simulink library "SADlibrary"  (R2020b)
settings: Solver=VariableStepAuto  StartTime=0.0  StopTime=10.0  RelTol=1e-3
libraries: vrlib x1, aerolibutil x1
settings Model: Creator=matteo  LastModifiedBy=matteo

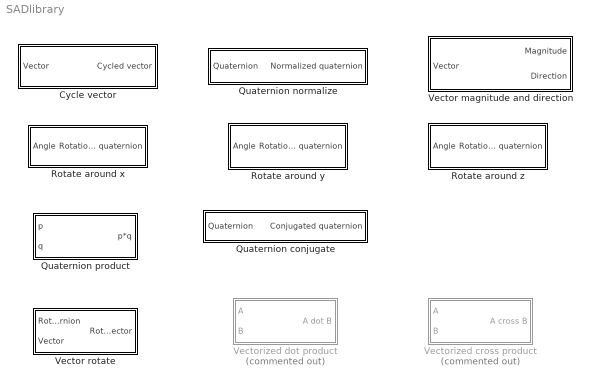
== system SADlibrary ==
  Cycle vector : Subsystem
  Quaternion conjugate : Subsystem
  Quaternion normalize : Subsystem
  Quaternion product : Subsystem
  Rotate around x : Subsystem
  Rotate around y : Subsystem
  Rotate around z : Subsystem
  Vector magnitude and direction : Subsystem
  Vector rotate : Subsystem
  Vectorized cross product : Subsystem  Commented=on
  Vectorized dot product : Subsystem  Commented=on

== system SADlibrary/Cycle vector ==
  Vector : Inport
  Demux : Demux  Outputs=2
  Mux : Mux  Inputs=2
  Cycled vector : Outport
  wires:
  Demux/1 -> Mux/2
  Mux/1 -> Cycled vector/1
  Vector/1 -> Demux/1
  Demux/2 -> Mux/1

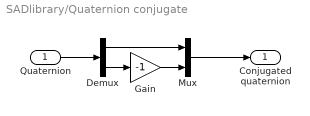
== system SADlibrary/Quaternion conjugate ==
  Quaternion : Inport
  Demux : Demux  Outputs=2
  Gain : Gain  Gain=-1
  Mux : Mux  Inputs=2
  Conjugated quaternion : Outport
  wires:
  Quaternion/1 -> Demux/1
  Demux/2 -> Gain/1
  Gain/1 -> Mux/2
  Demux/1 -> Mux/1
  Mux/1 -> Conjugated quaternion/1

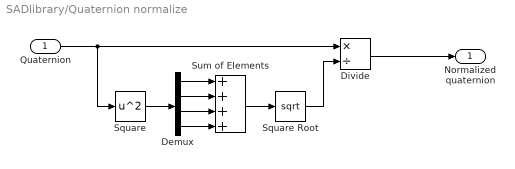
== system SADlibrary/Quaternion normalize ==
  Quaternion : Inport
  Demux : Demux
  Divide : Product  Inputs=*/
  Square : Math  Operator=square  SaturateOnIntegerOverflow=on
  Square Root : Sqrt  SaturateOnIntegerOverflow=on
  Sum of Elements : Sum  Inputs=++++
  Normalized quaternion : Outport
  wires:
  Quaternion/1 -> Divide/1, Square/1
  Square/1 -> Demux/1
  Demux/1 -> Sum of Elements/1
  Demux/2 -> Sum of Elements/2
  Demux/3 -> Sum of Elements/3
  Demux/4 -> Sum of Elements/4
  Sum of Elements/1 -> Square Root/1
  Square Root/1 -> Divide/2
  Divide/1 -> Normalized quaternion/1

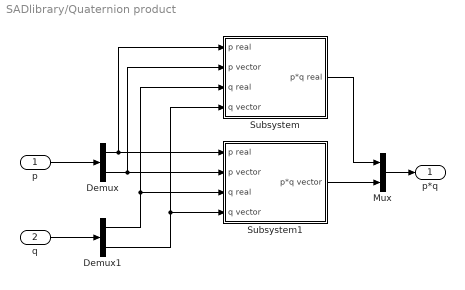
== system SADlibrary/Quaternion product ==
  p : Inport
  q : Inport  Port=2
  Demux : Demux  Outputs=2
  Demux1 : Demux  Outputs=2
  Mux : Mux  Inputs=2
  Subsystem : Subsystem
  Subsystem1 : Subsystem
  p*q : Outport
  wires:
  p/1 -> Demux/1
  q/1 -> Demux1/1
  Demux/1 -> Subsystem1/1(p real), Subsystem/1(p real)
  Demux1/1 -> Subsystem1/3(q real), Subsystem/3(q real)
  Demux/2 -> Subsystem1/2(p vector), Subsystem/2(p vector)
  Demux1/2 -> Subsystem1/4(q vector), Subsystem/4(q vector)
  Mux/1 -> p*q/1
  Subsystem/1(p*q real) -> Mux/1
  Subsystem1/1(p*q vector) -> Mux/2

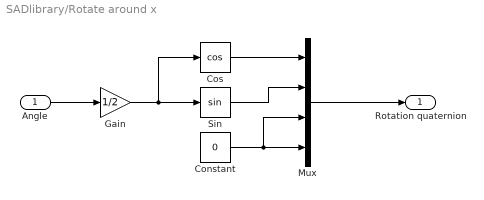
== system SADlibrary/Rotate around x ==
  Angle : Inport
  Constant : Constant  Value=0
  Cos : Trigonometry  Operator=cos
  Gain : Gain  Gain=1/2
  Mux : Mux
  Sin : Trigonometry
  Rotation quaternion : Outport
  wires:
  Sin/1 -> Mux/2
  Constant/1 -> Mux/3, Mux/4
  Angle/1 -> Gain/1
  Mux/1 -> Rotation quaternion/1
  Cos/1 -> Mux/1
  Gain/1 -> Cos/1, Sin/1

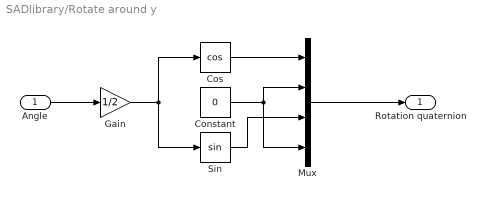
== system SADlibrary/Rotate around y ==
  Angle : Inport
  Constant : Constant  Value=0
  Cos : Trigonometry  Operator=cos
  Gain : Gain  Gain=1/2
  Mux : Mux
  Sin : Trigonometry
  Rotation quaternion : Outport
  wires:
  Cos/1 -> Mux/1
  Gain/1 -> Sin/1, Cos/1
  Constant/1 -> Mux/4, Mux/2
  Mux/1 -> Rotation quaternion/1
  Angle/1 -> Gain/1
  Sin/1 -> Mux/3

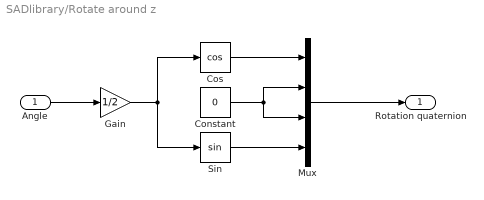
== system SADlibrary/Rotate around z ==
  Angle : Inport
  Constant : Constant  Value=0
  Cos : Trigonometry  Operator=cos
  Gain : Gain  Gain=1/2
  Mux : Mux
  Sin : Trigonometry
  Rotation quaternion : Outport
  wires:
  Angle/1 -> Gain/1
  Gain/1 -> Sin/1, Cos/1
  Constant/1 -> Mux/2, Mux/3
  Sin/1 -> Mux/4
  Cos/1 -> Mux/1
  Mux/1 -> Rotation quaternion/1

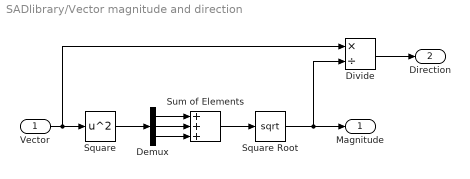
== system SADlibrary/Vector magnitude and direction ==
  Vector : Inport
  Demux : Demux  Outputs=3
  Divide : Product  Inputs=*/
  Square : Math  Operator=square  SaturateOnIntegerOverflow=on
  Square Root : Sqrt  SaturateOnIntegerOverflow=on
  Sum of Elements : Sum  Inputs=+++
  Magnitude : Outport
  Direction : Outport  Port=2
  wires:
  Vector/1 -> Divide/1, Square/1
  Demux/2 -> Sum of Elements/2
  Square/1 -> Demux/1
  Sum of Elements/1 -> Square Root/1
  Square Root/1 -> Divide/2, Magnitude/1
  Demux/3 -> Sum of Elements/3
  Demux/1 -> Sum of Elements/1
  Divide/1 -> Direction/1

== system SADlibrary/Vector rotate ==
  Rotation quaternion : Inport
  Vector : Inport  Port=2
  Quaternion Rotation : aerolibutil/Quaternion Rotation
  Rotated vector : Outport
  wires:
  Rotation quaternion/1 -> Quaternion Rotation/1
  Vector/1 -> Quaternion Rotation/2
  Quaternion Rotation/1 -> Rotated vector/1

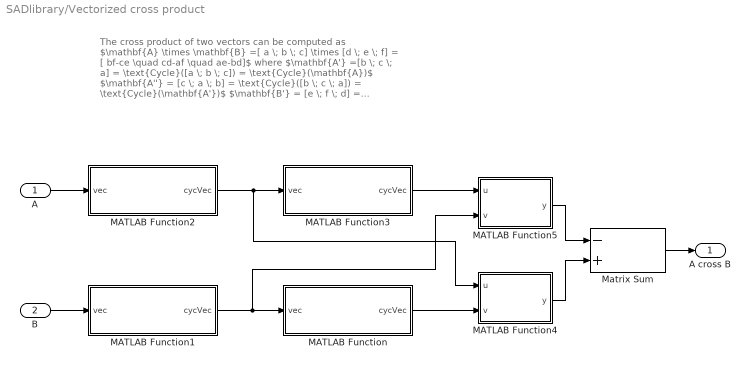
== system SADlibrary/Vectorized cross product ==
  note: The cross product of two vectors can be computed as
      | $\mathbf{A} \times \mathbf{B} =[ a \; b \; c] \times [d \; e \; f] = [ bf-ce \quad cd-af \quad ae-bd]$
      | where
      | $\mathbf{A'} =[b \; c \; a] = \text{Cycle}([a \; b \; c]) = \text{Cycle}(\mathbf{A})$
      | $\mathbf{A''} = [c \; a \; b] = \text{Cycle}([b \; c \; a]) = \text{Cycle}(\mathbf{A'})$
      | $\mathbf{B'} = [e \; f \; d] = \text{Cycle}([d \; e \; f] ) = \text{Cycle}(\mathbf{B})$
      | $\mathbf{B''} = [f \; d \; e] = \text{Cycle}([e \; f \; d] ) = \text{Cycle}(\mathbf{B'})$
      | so
      | $\mathbf{A} \times \mathbf{B} = \mathbf{A'} .* \mathbf{B''} - \mathbf{A''} .* \mathbf{B'}$
  A : Inport
  B : Inport  Port=2
  MATLAB Function : MATLAB Function  TreatAsAtomicUnit=on
  MATLAB Function1 : MATLAB Function  TreatAsAtomicUnit=on
  MATLAB Function2 : MATLAB Function  TreatAsAtomicUnit=on
  MATLAB Function3 : MATLAB Function  TreatAsAtomicUnit=on
  MATLAB Function4 : MATLAB Function  TreatAsAtomicUnit=on
  MATLAB Function5 : MATLAB Function  TreatAsAtomicUnit=on
  Matrix Sum : Sum  Inputs=-+
  A cross B : Outport
  wires:
  MATLAB Function2/1(cycVec) -> MATLAB Function4/1(u), MATLAB Function3/1(vec)
  MATLAB Function1/1(cycVec) -> MATLAB Function5/2(v), MATLAB Function/1(vec)
  MATLAB Function/1(cycVec) -> MATLAB Function4/2(v)
  MATLAB Function3/1(cycVec) -> MATLAB Function5/1(u)
  MATLAB Function4/1(y) -> Matrix Sum/2
  MATLAB Function5/1(y) -> Matrix Sum/1
  Matrix Sum/1 -> A cross B/1
  B/1 -> MATLAB Function1/1(vec)
  A/1 -> MATLAB Function2/1(vec)

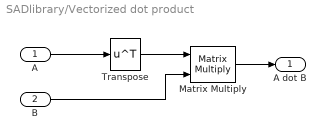
== system SADlibrary/Vectorized dot product ==
  A : Inport
  B : Inport  Port=2
  Matrix Multiply : Product  Multiplication=Matrix(*)
  Transpose : Math  Operator=transpose  SaturateOnIntegerOverflow=on
  A dot B : Outport
  wires:
  A/1 -> Transpose/1
  Transpose/1 -> Matrix Multiply/1
  B/1 -> Matrix Multiply/2
  Matrix Multiply/1 -> A dot B/1

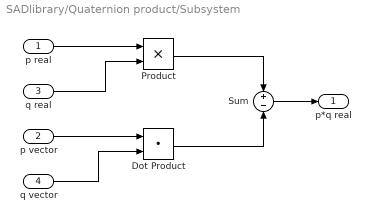
== system SADlibrary/Quaternion product/Subsystem ==
  p real : Inport
  p vector : Inport  Port=2
  q real : Inport  Port=3
  q vector : Inport  Port=4
  Dot Product : DotProduct  InputSameDT=on  OutDataTypeStr=Inherit: Inherit via internal rule
  Product : Product
  Sum : Sum  Inputs=+-
  p*q real : Outport
  wires:
  p vector/1 -> Dot Product/1
  q vector/1 -> Dot Product/2
  p real/1 -> Product/1
  q real/1 -> Product/2
  Product/1 -> Sum/1
  Dot Product/1 -> Sum/2
  Sum/1 -> p*q real/1

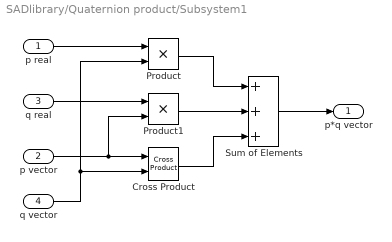
== system SADlibrary/Quaternion product/Subsystem1 ==
  p real : Inport
  p vector : Inport  Port=2
  q real : Inport  Port=3
  q vector : Inport  Port=4
  Cross Product : vrlib/Utilities/Cross Product
  Product : Product
  Product1 : Product
  Sum of Elements : Sum  Inputs=+++
  p*q vector : Outport
  wires:
  p real/1 -> Product/1
  p vector/1 -> Cross Product/1, Product1/2
  q vector/1 -> Cross Product/2, Product/2
  q real/1 -> Product1/1
  Product1/1 -> Sum of Elements/2
  Product/1 -> Sum of Elements/1
  Cross Product/1 -> Sum of Elements/3
  Sum of Elements/1 -> p*q vector/1

== matlab function SADlibrary/Vectorized cross product/MATLAB Function ==
  data: vec input; cycVec output
function cycVec = CycleRows(vec)

cycVec = circshift(vec,-1);

== matlab function SADlibrary/Vectorized cross product/MATLAB Function2 ==
  data: vec input; cycVec output
function cycVec = CycleRows(vec)

cycVec = circshift(vec,-1);

== matlab function SADlibrary/Vectorized cross product/MATLAB Function3 ==
  data: vec input; cycVec output
function cycVec = CycleRows(vec)

cycVec = circshift(vec,-1);

== matlab function SADlibrary/Vectorized cross product/MATLAB Function4 ==
  data: u input; y output; v input
function y = Product(u,v)

y = u.*v;

== matlab function SADlibrary/Vectorized cross product/MATLAB Function5 ==
  data: u input; y output; v input
function y = Product(u,v)

y = u.*v;

== matlab function SADlibrary/Vectorized cross product/MATLAB Function1 ==
  data: vec input; cycVec output
function cycVec = CycleRows(vec)

cycVec = circshift(vec,-1);
